simulink model "mrac_ZG"  (R2023a)
settings: Solver=ode5  StartTime=0.0  StopTime=60  FixedStep=0.001  RelTol=1e-3
values from neighbouring files (symbols this model uses):
  A_ref = app.RefModelAField.Value    [MRACApp.m]    (also in MRAC_Main_Script.m = input('A matrisi: '); mrac_combined.m = [0 1; -1 -1.4])
  B_ref = app.RefModelBField.Value    [MRACApp.m]    (also in MRAC_Main_Script.m = input('B matrisi: '); mrac_combined.m = [0; 1])
  C_ref = app.RefModelCField.Value    [MRACApp.m]    (also in MRAC_Main_Script.m = input('C matrisi: '); mrac_combined.m = eye(2))
  D_ref = app.RefModelDField.Value    [MRACApp.m]    (also in MRAC_Main_Script.m = input('D matrisi: '); mrac_combined.m = [0; 0])
undefined symbols (not defined in the file or in its folder): As, Bs, Cs, Ds
settings Model: Creator=merve  LastModifiedBy=merve
settings DataIOCC: ReturnWorkspaceOutputs=off

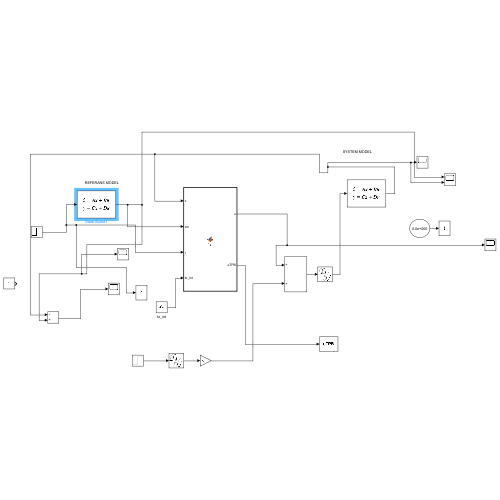
[thumbnail: Simulink's stored preview of the top-level diagram]
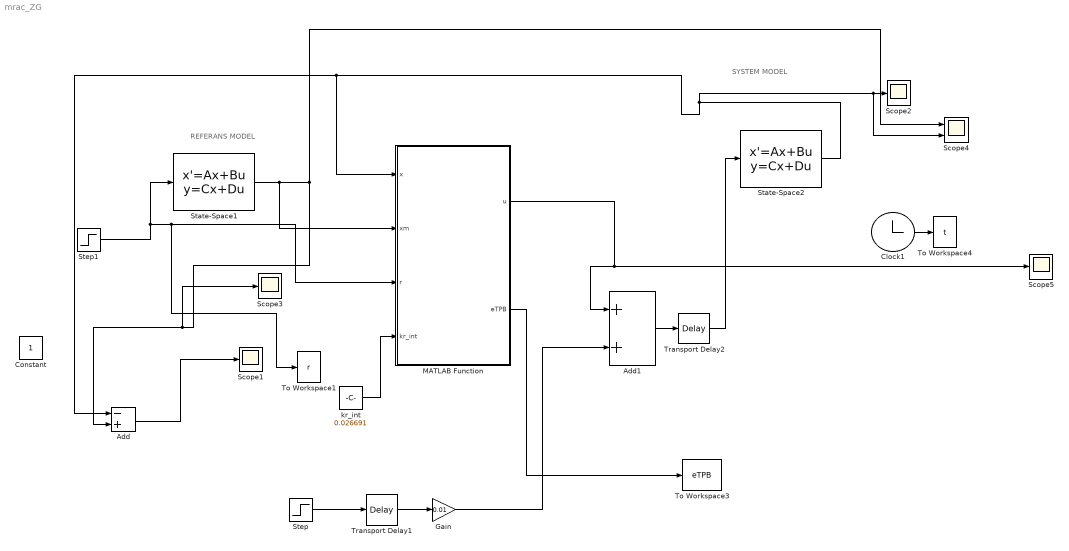
== system mrac_ZG ==
  note: REFERANS MODEL
  note: SYSTEM MODEL
  Add : Sum  Inputs=-+
  Add1 : Sum
  Clock1 : Clock
  Constant : Constant
  Gain : Gain  Gain=0.01
  MATLAB Function : MATLAB Function  TreatAsAtomicUnit=on
  Scope{1..3,5} (4 alike) : Scope
  Scope4 : Scope  NumInputPorts=2
  State-Space1 : StateSpace  A=A_ref  B=B_ref  C=C_ref  D=D_ref  InitialCondition=0
  State-Space2 : StateSpace  A=As  B=Bs  C=Cs  D=Ds  InitialCondition=0
  Step : Step  SampleTime=0
  Step1 : Step  SampleTime=0
  To Workspace1 : ToWorkspace  VariableName=r  SampleTime=-1
  To Workspace3 : ToWorkspace  VariableName=eTPB  SampleTime=-1
  To Workspace4 : ToWorkspace  VariableName=t  SampleTime=-1
  Transport Delay1 : TransportDelay  DelayTime=5
  Transport Delay2 : TransportDelay  DelayTime=0.2
  kr_int : Constant  Value=0.026691  SampleTime=0.001
  wires:
  Step1/1 -> State-Space1/1, To Workspace1/1, MATLAB Function/3(r)
  State-Space2/1 -> Scope4/2, Scope2/1, MATLAB Function/1(x), Add/1
  Add/1 -> Scope1/1
  Clock1/1 -> To Workspace4/1
  State-Space1/1 -> MATLAB Function/2(xm), Scope4/1, Scope3/1, Add/2
  MATLAB Function/1(u) -> Add1/1, Scope5/1
  Step/1 -> Transport Delay1/1
  Transport Delay1/1 -> Gain/1
  Add1/1 -> Transport Delay2/1
  Gain/1 -> Add1/2
  Transport Delay2/1 -> State-Space2/1
  MATLAB Function/2(eTPB) -> To Workspace3/1
  kr_int/1 -> MATLAB Function/4(kr_int)

== matlab function mrac_ZG/MATLAB Function ==
  settings: updateMethod=DISCRETE
  data: x input; xm input; u output; r input; kr_int input; eTPB output
% HT-MRAK Kontrol Yapısı – MATLAB Function
function [u,eTPB]  = fcn(x, xm, r,kr_int)

    %% Sabitler
    P = [2.799 3.125;
         3.125 6.359];
    B = [0; 1];
   
    k1 = 1;      % hata telafi kazancı
    dt = 0.001;  % örnekleme süresi
   

    %% Hata
    e = x - xm; % takip hatası
 eTPB = e' * P * B;    % skalar
    %% Kontrol sinyali: u = kr*r - k1*BᵗPe
    u_a = kr_int * r;                     % adaptif parça
    u_c = -k1 * (B' * P * e);             % hata telafi parçası
    u = u_a + u_c;                        % toplam kontrol sinyali

   
end
